simulink model "Throttle_Map"  (R2022b)
settings: Solver=VariableStepAuto  StartTime=0.0  StopTime=10.0  RelTol=1e-3
undefined symbols (not defined in the file or in its folder): k_grid_max, k_grid_min, rpm_sweep_min, voltage_sweep_min
libraries: simulink x1
settings Model: Creator=Inver  LastModifiedBy=Inver

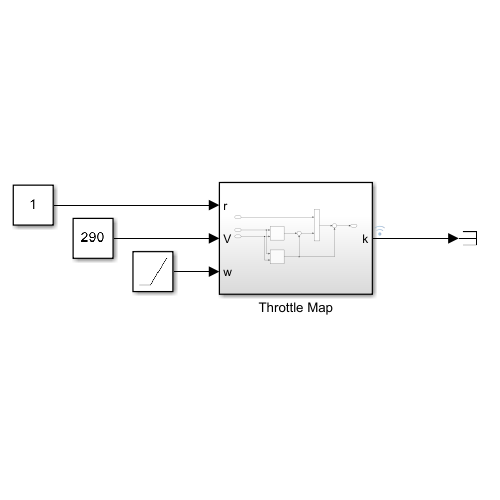
[thumbnail: Simulink's stored preview of the top-level diagram]
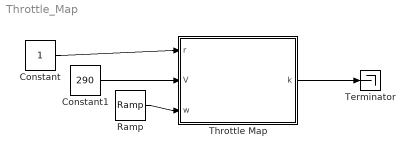
== system Throttle_Map ==
  Constant : Constant
  Constant1 : Constant  Value=290
  Ramp : simulink/Sources/Ramp  slope=100  start=0  InitialOutput=0
  Terminator : Terminator
  Throttle Map : Subsystem
  wires:
  Throttle Map/1(k) -> Terminator/1
  Constant/1 -> Throttle Map/1(r)
  Constant1/1 -> Throttle Map/2(V)
  Ramp/1 -> Throttle Map/3(w)

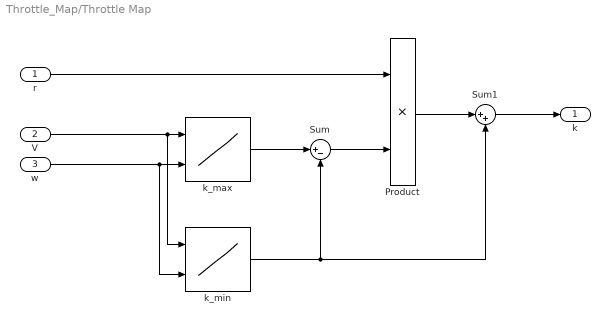
== system Throttle_Map/Throttle Map ==
  r : Inport
  V : Inport  Port=2
  w : Inport  Port=3
  Product : Product
  Sum : Sum  Inputs=|+-
  Sum1 : Sum  Inputs=|++
  k_max : Lookup_n-D  LookupTableObject=''  BreakpointsForDimension1=voltage_sweep_min  BreakpointsForDimension2=rpm_sweep_min  BreakpointsForDimension1FirstPoint=10  BreakpointsForDimension2FirstPoint=10  BreakpointsForDimension1Spacing=12  BreakpointsForDimension2Spacing=12  IndexSearchMethod=Evenly spaced points  Table=k_grid_max  ExtrapMethod=Clip  DiagnosticForOutOfRangeInput=Error  InternalRulePriority=Speed  RndMeth=Simplest
      settings: InputPortMap=u0,u1
  k_min : Lookup_n-D  LookupTableObject=''  BreakpointsForDimension1=voltage_sweep_min  BreakpointsForDimension2=rpm_sweep_min  BreakpointsForDimension1FirstPoint=10  BreakpointsForDimension2FirstPoint=10  BreakpointsForDimension1Spacing=12  BreakpointsForDimension2Spacing=12  IndexSearchMethod=Evenly spaced points  Table=k_grid_min  ExtrapMethod=Clip  DiagnosticForOutOfRangeInput=Error  InternalRulePriority=Speed  RndMeth=Simplest
      settings: InputPortMap=u0,u1
  k : Outport
  wires:
  Sum/1 -> Product/2
  k_max/1 -> Sum/1
  V/1 -> k_min/1, k_max/1
  r/1 -> Product/1
  k_min/1 -> Sum1/2, Sum/2
  w/1 -> k_min/2, k_max/2
  Product/1 -> Sum1/1
  Sum1/1 -> k/1
